simulink model "Interpretation_Unit"  (R2019a)
settings: Solver=ode2  StartTime=0.0  StopTime=inf  FixedStep=0.002  RelTol=1e-3  EnableMultiTasking=on
libraries: simulink x10, quarc_library x4
settings Model: Creator=User  LastModifiedBy=mbohra
settings SolverCC: PositivePriorityOrder=on
settings DataIOCC: ReturnWorkspaceOutputs=off
settings DebuggingCC: PregeneratedLibrarySubsystemCodeDiagnostic=none  ArithmeticOperatorsInVariantConditions=warning
settings SFSimCC: SimUseLocalCustomCode=off
settings RTWCC: SystemTargetFile=quarc_linux_nvidia.tlc  TemplateMakefile=quarc_linux_nvidia_tmf  Description=QUARC Linux Nvidia Target  RTWUseLocalCustomCode=off
settings STFCustomTargetCC: TargetLibSuffix=.a  TargetPreCompLibLocation=C:\PROGRA~3\QUARC\lib\2019a\LINUX_~1\release  TargetLangStandard=C99 (ISO)  ConcurrentExecutionCompliant=on  SystemTargetFile=quarc_linux_nvidia.tlc
settings GRTTargetCC: TargetLibSuffix=.a  TargetPreCompLibLocation=C:\PROGRA~3\QUARC\lib\2019a\LINUX_~1\release  ParMdlRefBuildCompliant=off  CompOptLevelCompliant=off  CombineOutputUpdateFcns=off  MatFileLogging=off  CPPClassGenCompliant=off  GRTInterface=on  UseToolchainInfoCompliant=off  ExtMode=on  ExtModeMexFile=quarc_comm  ExtModeMexArgs='-w -d /tmp -uri %u'

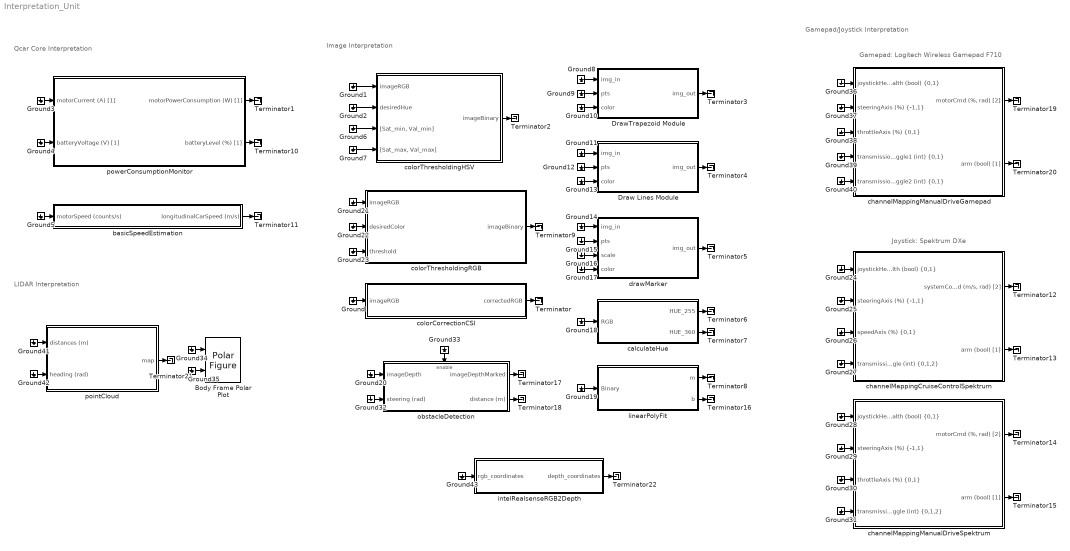
== system Interpretation_Unit ==
  note: LIDAR Interpretation
  note: Gamepad/Joystick Interpretation
  note: Image Interpretation
  note: Qcar Core Interpretation
  note: Gamepad: Logitech Wireless Gamepad F710
  note: Joystick: Spektrum DXe
  Body Frame Polar Plot : quarc_library/Sinks/Figures/Polar Figure  figure_mode=Use figure window  figure_tag=figure1  axes_tag=axes1  plot_mode=Frame-based  minimum_rho=0  maximum_rho=1  minimum_theta=0  maximum_theta=360  zero_location=right  direction=counterclockwise  buffer_size=1000  update_rate=1  sample_time=-1  initial_position="-1919             41           1920          990.4"  initial_visibility=off  line1_style=None  line1_width=0.5  line1_color=[0 0.4470 0.7410]  marker1=Circle (o)  marker1_size=1  marker1_edge_color=[0 0.447059 0.741176]  marker1_face_color=[0 0.447059 0.741176]  line2_style=Solid line (-)  line2_width=0.5  line2_color=[0.85098 0.32549 0.0980392]  marker2=None  marker2_size=6  marker2_edge_color=[0.85098 0.32549 0.0980392]  marker2_face_color=[0.85098 0.32549 0.0980392]  line3_style=Solid line (-)  line3_width=0.5  line3_color=[0.929412 0.694118 0.12549]  marker3=None  marker3_size=6  marker3_edge_color=[0.929412 0.694118 0.12549]  marker3_face_color=[0.929412 0.694118 0.12549]  line4_style=Solid line (-)  line4_width=0.5  line4_color=[0.494118 0.184314 0.556863]  marker4=None  marker4_size=6  marker4_edge_color=[0.494118 0.184314 0.556863]  marker4_face_color=[0.494118 0.184314 0.556863]  line5_style=Solid line (-)  line5_width=0.5  line5_color=[0.466667 0.67451 0.188235]  marker5=None  marker5_size=6  marker5_edge_color=[0.466667 0.67451 0.188235]  marker5_face_color=[0.466667 0.67451 0.188235]
      settings: SourceProductName=QUARC Targets
  Draw Lines Module : MATLAB Function  TreatAsAtomicUnit=on
  DrawTrapezoid Module : MATLAB Function  TreatAsAtomicUnit=on
  Ground{,1..43} (44 alike) : Ground
  Terminator{,1..22} (23 alike) : Terminator
  basicSpeedEstimation : Subsystem
  calculateHue : MATLAB Function  TreatAsAtomicUnit=on
  channelMappingCruiseControlSpektrum : Subsystem
  channelMappingManualDriveGamepad : Subsystem
  channelMappingManualDriveSpektrum : Subsystem
  colorCorrectionCSI : Subsystem
  colorThresholdingHSV : Subsystem
  colorThresholdingRGB : Subsystem
  drawMarker : MATLAB Function  TreatAsAtomicUnit=on
  intelRealsenseRGB2Depth : MATLAB Function  TreatAsAtomicUnit=on
  linearPolyFit : MATLAB Function  TreatAsAtomicUnit=on
  obstacleDetection : Subsystem
  pointCloud : Subsystem
  powerConsumptionMonitor : Subsystem
  wires:
  Ground23/1 -> colorThresholdingRGB/3("threshold ")
  basicSpeedEstimation/1(longitudinalCarSpeed (m/s)) -> Terminator11/1
  Ground18/1 -> calculateHue/1(RGB)
  calculateHue/1(HUE_255) -> Terminator6/1
  Ground22/1 -> colorThresholdingRGB/2(desiredColor)
  Ground5/1 -> basicSpeedEstimation/1(motorSpeed (counts/s))
  Ground1/1 -> colorThresholdingHSV/1(imageRGB)
  Ground8/1 -> DrawTrapezoid Module/1(img_in)
  Ground3/1 -> powerConsumptionMonitor/1(motorCurrent (A) [1])
  Ground14/1 -> drawMarker/1(img_in)
  Ground11/1 -> Draw Lines Module/1(img_in)
  Ground13/1 -> Draw Lines Module/3(color)
  powerConsumptionMonitor/2(batteryLevel (%) [1]) -> Terminator10/1
  colorThresholdingHSV/1(imageBinary) -> Terminator2/1
  powerConsumptionMonitor/1(motorPowerConsumption (W) [1]) -> Terminator1/1
  Ground16/1 -> drawMarker/3(scale)
  Ground7/1 -> colorThresholdingHSV/4("[Sat_max, Val_max]")
  Ground9/1 -> DrawTrapezoid Module/2(pts)
  Ground2/1 -> colorThresholdingHSV/2(desiredHue)
  Ground10/1 -> DrawTrapezoid Module/3(color)
  Ground15/1 -> drawMarker/2(pts)
  Ground12/1 -> Draw Lines Module/2(pts)
  Ground4/1 -> powerConsumptionMonitor/2(batteryVoltage (V) [1])
  Draw Lines Module/1(img_out) -> Terminator4/1
  colorThresholdingRGB/1(imageBinary) -> Terminator9/1
  Ground21/1 -> colorThresholdingRGB/1(imageRGB)
  DrawTrapezoid Module/1(img_out) -> Terminator3/1
  drawMarker/1(img_out) -> Terminator5/1
  colorCorrectionCSI/1(correctedRGB) -> Terminator/1
  Ground6/1 -> colorThresholdingHSV/3("[Sat_min, Val_min]")
  Ground17/1 -> drawMarker/4(color)
  calculateHue/2(HUE_360) -> Terminator7/1
  Ground/1 -> colorCorrectionCSI/1(imageRGB)
  channelMappingManualDriveSpektrum/2(arm (bool) [1]) -> Terminator15/1
  Ground25/1 -> channelMappingCruiseControlSpektrum/2("steeringAxis (%) {-1,1}")
  channelMappingCruiseControlSpektrum/2(arm (bool) [1]) -> Terminator13/1
  Ground29/1 -> channelMappingManualDriveSpektrum/2("steeringAxis (%) {-1,1}")
  channelMappingManualDriveSpektrum/1("motorCmd (%, rad) [2]") -> Terminator14/1
  Ground27/1 -> channelMappingCruiseControlSpektrum/4("transmissionToggle (int) {0,1,2}")
  Ground30/1 -> channelMappingManualDriveSpektrum/3("throttleAxis (%) {0,1}")
  Ground26/1 -> channelMappingCruiseControlSpektrum/3("speedAxis (%) {0,1}")
  Ground28/1 -> channelMappingManualDriveSpektrum/1("joystickHealth (bool) {0,1}")
  channelMappingCruiseControlSpektrum/1("systemCommand (m/s, rad) [2]") -> Terminator12/1
  Ground31/1 -> channelMappingManualDriveSpektrum/4("transmissionToggle (int) {0,1,2}")
  Ground24/1 -> channelMappingCruiseControlSpektrum/1("joystickHealth (bool) {0,1}")
  Ground34/1 -> Body Frame Polar Plot/1
  Ground35/1 -> Body Frame Polar Plot/2
  Ground36/1 -> channelMappingManualDriveGamepad/1("joystickHealth (bool) {0,1}")
  Ground37/1 -> channelMappingManualDriveGamepad/2("steeringAxis (%) {-1,1}")
  Ground38/1 -> channelMappingManualDriveGamepad/3("throttleAxis (%) {0,1}")
  Ground39/1 -> channelMappingManualDriveGamepad/4("transmissionToggle1 (int) {0,1}")
  Ground40/1 -> channelMappingManualDriveGamepad/5("transmissionToggle2 (int) {0,1}")
  channelMappingManualDriveGamepad/1("motorCmd (%, rad) [2]") -> Terminator19/1
  channelMappingManualDriveGamepad/2(arm (bool) [1]) -> Terminator20/1
  Ground41/1 -> pointCloud/1(distances (m))
  Ground42/1 -> pointCloud/2(heading (rad))
  pointCloud/1(map) -> Terminator21/1
  Ground19/1 -> linearPolyFit/1(Binary)
  linearPolyFit/1(m) -> Terminator8/1
  linearPolyFit/2(b) -> Terminator16/1
  Ground20/1 -> obstacleDetection/1(imageDepth)
  Ground32/1 -> obstacleDetection/2(steering (rad))
  obstacleDetection/1(imageDepthMarked) -> Terminator17/1
  obstacleDetection/2(distance (m)) -> Terminator18/1
  Ground33/1 -> obstacleDetection/Enable
  Ground43/1 -> intelRealsenseRGB2Depth/1(rgb_coordinates)
  intelRealsenseRGB2Depth/1(depth_coordinates) -> Terminator22/1

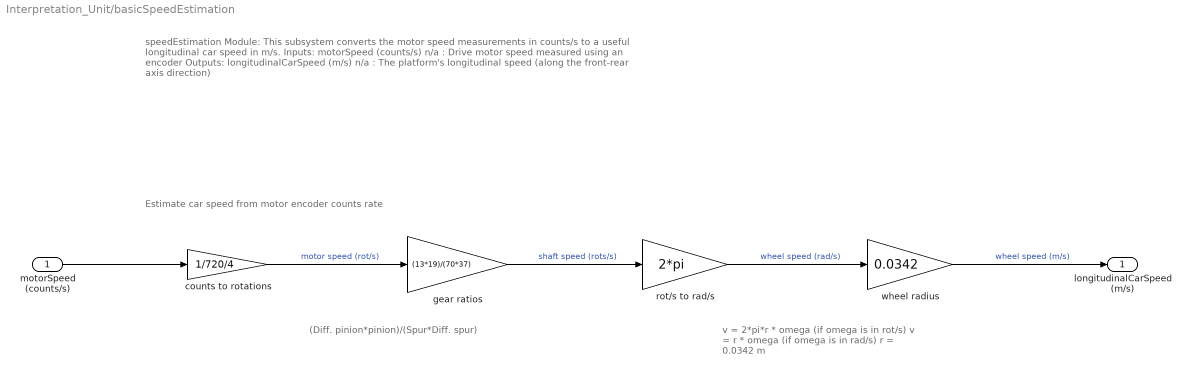
== system Interpretation_Unit/basicSpeedEstimation ==
  note: Estimate car speed from motor encoder counts rate
  note: v = 2*pi*r * omega (if omega is in rot/s)
      | v = r * omega (if omega is in rad/s)
      | r = 0.0342 m
  note: (Diff. pinion*pinion)/(Spur*Diff. spur)
  note: speedEstimation Module:
      |
      | This subsystem converts the motor speed measurements in counts/s to a useful longitudinal car speed in m/s.
      |
      | Inputs:
      | motorSpeed (counts/s) n/a : Drive motor speed measured using an encoder
      |
      | Outputs:
      | longitudinalCarSpeed (m/s) n/a : The platform's longitudinal speed (along the front-rear axis direction)
  motorSpeed (counts/s) : Inport
  counts to rotations : Gain  Gain=1/720/4
  gear ratios : Gain  Gain=(13*19)/(70*37)
  rot/s to rad/s : Gain  Gain=2*pi
  wheel radius : Gain  Gain=0.0342
  longitudinalCarSpeed (m/s) : Outport
  wires:
  motorSpeed (counts/s)/1 -> counts to rotations/1
  rot/s to rad/s/1 -> wheel radius/1  "wheel speed (rad/s)"
  counts to rotations/1 -> gear ratios/1  "motor speed (rot/s)"
  wheel radius/1 -> longitudinalCarSpeed (m/s)/1  "wheel speed (m/s)"
  gear ratios/1 -> rot/s to rad/s/1  "shaft speed (rots/s)"

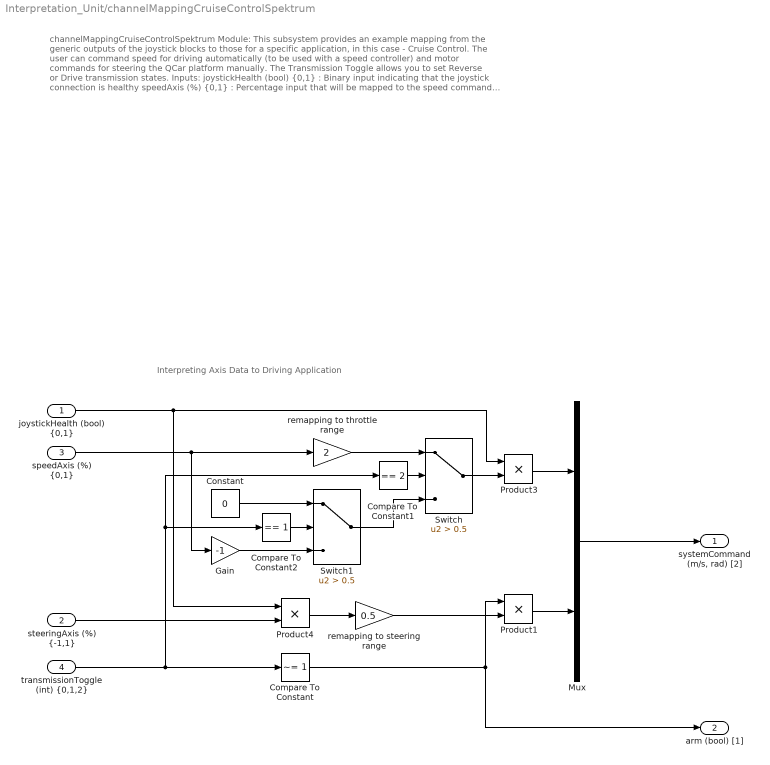
== system Interpretation_Unit/channelMappingCruiseControlSpektrum ==
  note: Interpreting Axis Data to Driving Application
  note: channelMappingCruiseControlSpektrum Module:
      |
      | This subsystem provides an example mapping from the generic outputs of the joystick blocks to those for a specific application, in this case - Cruise Control. The user can command speed for driving automatically (to be used with a speed controller) and motor commands for steering the QCar platform manually. The Transmission Toggle allows you to set Reverse or Drive transmission states.
      |
      | Inputs:
      | joystickHealth (bool) {0,1} : Binary input indicating that the joystick connection is healthy
      | speedAxis (%) {0,1} : Percentage input that will be mapped to the speed command
      | steeringAxis (%) {-1,1} : Signed percentage input that will be mapped to steering
      | transmissionToggle (int) {0,1,2} : 3-state input that will decide the Reverse/Park/Drive states
      |
      | Outputs:
      | systemCommand (m/s, rad) n/a : Vector output for the speed command (m/s) as well as steering command (in rad)
      | arm (bool) {0,1} : Binary output indicating status (armed or disarmed)
      |
      | Usage:
      | 1. When the Transmission Toggle input
      | a. reads 0 or 2, the Arm output will be high (1), which is the Armed state.
      | b. reads 1, the Arm output will be low (0), which is the Disarmed state.
      | 2. In addition, the Transmission Toggle input
      | a. reading 0 is the Reverse state, and the Speed Command will range from 0 m/s to -1 m/s, spinning the wheels backwards.
      | b. reading 1 is the Park state, and the Speed Command will be zero.
      | c. reading 2 is the Drive state, and the Speed Command will range from 0 m/s to 2 m/s, spinning the wheels forwards.
  "joystickHealth (bool) {0,1}" : Inport
  "steeringAxis (%) {-1,1}" : Inport  Port=2
  "speedAxis (%) {0,1}" : Inport  Port=3
  "transmissionToggle (int) {0,1,2}" : Inport  Port=4
  " remapping to steering range " : Gain  Gain=0.5
  Compare To Constant : simulink/Logic and Bit Operations/Compare To Constant  relop=~=  const=1  OutDataTypeStr=boolean
  Compare To Constant1 : simulink/Logic and Bit Operations/Compare To Constant  relop===  const=2  OutDataTypeStr=boolean
  Compare To Constant2 : simulink/Logic and Bit Operations/Compare To Constant  relop===  const=1  OutDataTypeStr=boolean
  Constant : Constant  Value=0
  Gain : Gain  Gain=-1
  Mux : Mux  Inputs=2
  Product1 : Product
  Product3 : Product
  Product4 : Product
  Switch : Switch  Criteria=u2 > Threshold  Threshold=0.5
  Switch1 : Switch  Criteria=u2 > Threshold  Threshold=0.5
  remapping to throttle range : Gain  Gain=2
  "systemCommand (m/s, rad) [2]" : Outport
  arm (bool) [1] : Outport  Port=2
  wires:
  Switch1/1 -> Switch/3
  Gain/1 -> Switch1/3
  Compare To Constant/1 -> arm (bool) [1]/1, Product1/1
  Compare To Constant2/1 -> Switch1/2
  Constant/1 -> Switch1/1
  "joystickHealth (bool) {0,1}"/1 -> Product3/1, Product4/1
  Compare To Constant1/1 -> Switch/2
  Product4/1 -> " remapping to steering range "/1
  remapping to throttle range/1 -> Switch/1
  "transmissionToggle (int) {0,1,2}"/1 -> Compare To Constant2/1, Compare To Constant1/1, Compare To Constant/1
  Product3/1 -> Mux/1
  "speedAxis (%) {0,1}"/1 -> Gain/1, remapping to throttle range/1
  " remapping to steering range "/1 -> Product1/2
  "steeringAxis (%) {-1,1}"/1 -> Product4/2
  Product1/1 -> Mux/2
  Mux/1 -> "systemCommand (m/s, rad) [2]"/1
  Switch/1 -> Product3/2

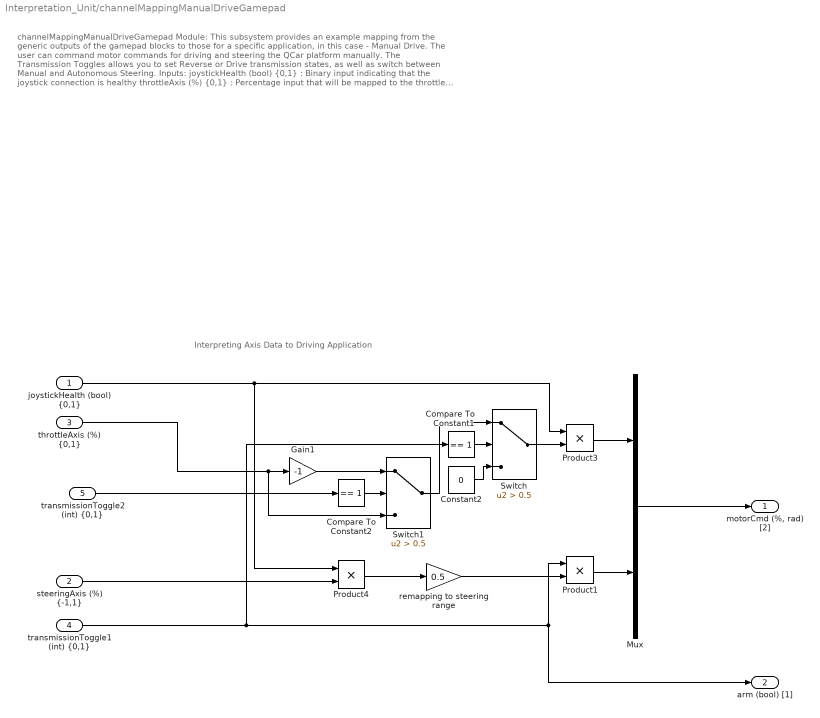
== system Interpretation_Unit/channelMappingManualDriveGamepad ==
  note: Interpreting Axis Data to Driving Application
  note: channelMappingManualDriveGamepad Module:
      |
      | This subsystem provides an example mapping from the generic outputs of the gamepad blocks to those for a specific application, in this case - Manual Drive. The user can command motor commands for driving and steering the QCar platform manually. The Transmission Toggles allows you to set Reverse or Drive transmission states, as well as switch between Manual and Autonomous Steering.
      |
      | Inputs:
      | joystickHealth (bool) {0,1} : Binary input indicating that the joystick connection is healthy
      | throttleAxis (%) {0,1} : Percentage input that will be mapped to the throttle command
      | steeringAxis (%) {-1,1} : Signed percentage input that will be mapped to steering
      | transmissionToggle1 (int) {0,1} : 2-state input that will decide the Park/Engage State
      | transmissionToggle2 (int) {0, 1} : 2-state input that will decide the Reverse/Drive State
      |
      | Outputs:
      | motorCmd (%, rad) n/a : Vector output for the motor drive command (percentage throttle) as well as steering command (in rad)
      | arm (bool) {0,1} : Binary output indicating status (armed or disarmed)
      |
      | Usage:
      | 1. When the Transmission Toggle 1 input
      | a. reads 1, the Arm output will be high (1), which is the Armed state.
      | b. reads 0, the Arm output will be low (0), which is the Disarmed state.
      | 2. In addition, the Transmission Toggle 2 input
      | a. reading 0 is the Drive state, and the Motor Cmd for the throttle will range from 0 to 100%, spinning the wheels forwards.
      | b. reading 1 is the Reverse state, and the Motor Cmd for the throttle will range from 0 to -100%, spinning the wheels backwards.
  "joystickHealth (bool) {0,1}" : Inport
  "steeringAxis (%) {-1,1}" : Inport  Port=2
  "throttleAxis (%) {0,1}" : Inport  Port=3
  "transmissionToggle1 (int) {0,1}" : Inport  Port=4
  "transmissionToggle2 (int) {0,1}" : Inport  Port=5
  " remapping to steering range " : Gain  Gain=0.5
  Compare To Constant1 : simulink/Logic and Bit Operations/Compare To Constant  relop===  const=1  OutDataTypeStr=boolean
  Compare To Constant2 : simulink/Logic and Bit Operations/Compare To Constant  relop===  const=1  OutDataTypeStr=boolean
  Constant2 : Constant  Value=0
  Gain1 : Gain  Gain=-1
  Mux : Mux  Inputs=2
  Product1 : Product
  Product3 : Product
  Product4 : Product
  Switch : Switch  Criteria=u2 > Threshold  Threshold=0.5
  Switch1 : Switch  Criteria=u2 > Threshold  Threshold=0.5
  "motorCmd (%, rad) [2]" : Outport
  arm (bool) [1] : Outport  Port=2
  wires:
  Gain1/1 -> Switch1/1
  "transmissionToggle2 (int) {0,1}"/1 -> Compare To Constant2/1
  Constant2/1 -> Switch/3
  Switch1/1 -> Switch/1
  Compare To Constant2/1 -> Switch1/2
  Mux/1 -> "motorCmd (%, rad) [2]"/1
  "throttleAxis (%) {0,1}"/1 -> Gain1/1, Switch1/3
  Product4/1 -> " remapping to steering range "/1
  " remapping to steering range "/1 -> Product1/2
  Product3/1 -> Mux/1
  "transmissionToggle1 (int) {0,1}"/1 -> arm (bool) [1]/1, Product1/1, Compare To Constant1/1
  "joystickHealth (bool) {0,1}"/1 -> Product3/1, Product4/1
  "steeringAxis (%) {-1,1}"/1 -> Product4/2
  Compare To Constant1/1 -> Switch/2
  Product1/1 -> Mux/2
  Switch/1 -> Product3/2

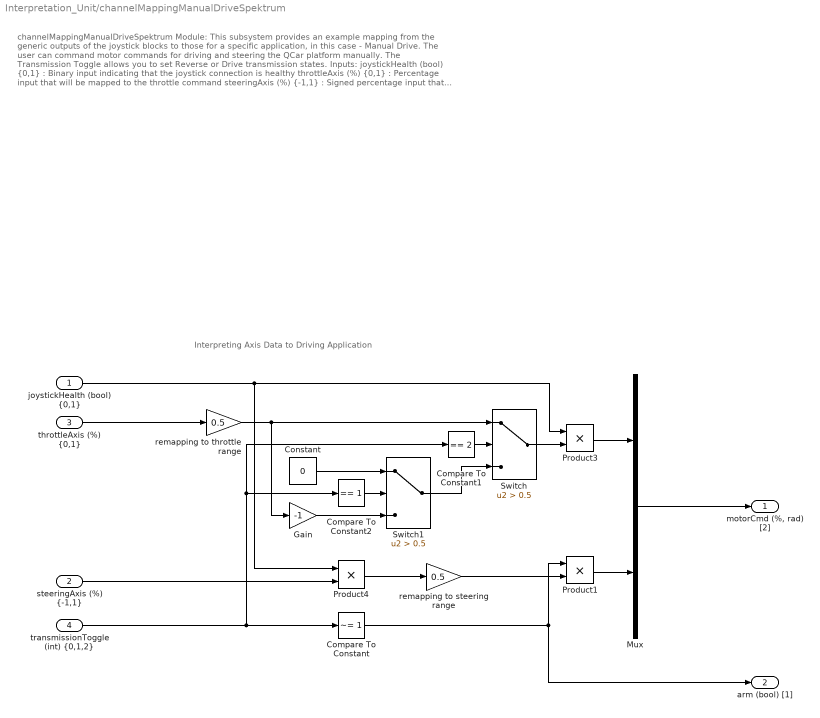
== system Interpretation_Unit/channelMappingManualDriveSpektrum ==
  note: Interpreting Axis Data to Driving Application
  note: channelMappingManualDriveSpektrum Module:
      |
      | This subsystem provides an example mapping from the generic outputs of the joystick blocks to those for a specific application, in this case - Manual Drive. The user can command motor commands for driving and steering the QCar platform manually. The Transmission Toggle allows you to set Reverse or Drive transmission states.
      |
      | Inputs:
      | joystickHealth (bool) {0,1} : Binary input indicating that the joystick connection is healthy
      | throttleAxis (%) {0,1} : Percentage input that will be mapped to the throttle command
      | steeringAxis (%) {-1,1} : Signed percentage input that will be mapped to steering
      | transmissionToggle (int) {0,1,2} : 3-state input that will decide the Reverse/Park/Drive states
      |
      | Outputs:
      | motorCmd (%, rad) n/a : Vector output for the motor drive command (percentage throttle) as well as steering command (in rad)
      | arm (bool) {0,1} : Binary output indicating status (armed or disarmed)
      |
      | Usage:
      | 1. When the Transmission Toggle input
      | a. reads 0 or 2, the Arm output will be high (1), which is the Armed state.
      | b. reads 1, the Arm output will be low (0), which is the Disarmed state.
      | 2. In addition, the Transmission Toggle input
      | a. reading 0 is the Reverse state, and the Motor Cmd for the throttle will range from 0 to -50%, spinning the wheels backwards.
      | b. reading 1 is the Park state, and the Motor Cmd for the throttle will be zero.
      | c. reading 2 is the Drive state, and the Motor Cmd for the throttle will range from 0 to 50%, spinning the wheels forwards.
  "joystickHealth (bool) {0,1}" : Inport
  "steeringAxis (%) {-1,1}" : Inport  Port=2
  "throttleAxis (%) {0,1}" : Inport  Port=3
  "transmissionToggle (int) {0,1,2}" : Inport  Port=4
  " remapping to steering range " : Gain  Gain=0.5
  " remapping to throttle range" : Gain  Gain=0.5
  Compare To Constant : simulink/Logic and Bit Operations/Compare To Constant  relop=~=  const=1  OutDataTypeStr=boolean
  Compare To Constant1 : simulink/Logic and Bit Operations/Compare To Constant  relop===  const=2  OutDataTypeStr=boolean
  Compare To Constant2 : simulink/Logic and Bit Operations/Compare To Constant  relop===  const=1  OutDataTypeStr=boolean
  Constant : Constant  Value=0
  Gain : Gain  Gain=-1
  Mux : Mux  Inputs=2
  Product1 : Product
  Product3 : Product
  Product4 : Product
  Switch : Switch  Criteria=u2 > Threshold  Threshold=0.5
  Switch1 : Switch  Criteria=u2 > Threshold  Threshold=0.5
  "motorCmd (%, rad) [2]" : Outport
  arm (bool) [1] : Outport  Port=2
  wires:
  " remapping to throttle range"/1 -> Switch/1, Gain/1
  Constant/1 -> Switch1/1
  Compare To Constant2/1 -> Switch1/2
  Mux/1 -> "motorCmd (%, rad) [2]"/1
  Gain/1 -> Switch1/3
  Product4/1 -> " remapping to steering range "/1
  " remapping to steering range "/1 -> Product1/2
  Product3/1 -> Mux/1
  Compare To Constant/1 -> arm (bool) [1]/1, Product1/1
  "throttleAxis (%) {0,1}"/1 -> " remapping to throttle range"/1
  Switch1/1 -> Switch/3
  "joystickHealth (bool) {0,1}"/1 -> Product3/1, Product4/1
  "steeringAxis (%) {-1,1}"/1 -> Product4/2
  Compare To Constant1/1 -> Switch/2
  "transmissionToggle (int) {0,1,2}"/1 -> Compare To Constant2/1, Compare To Constant1/1, Compare To Constant/1
  Product1/1 -> Mux/2
  Switch/1 -> Product3/2

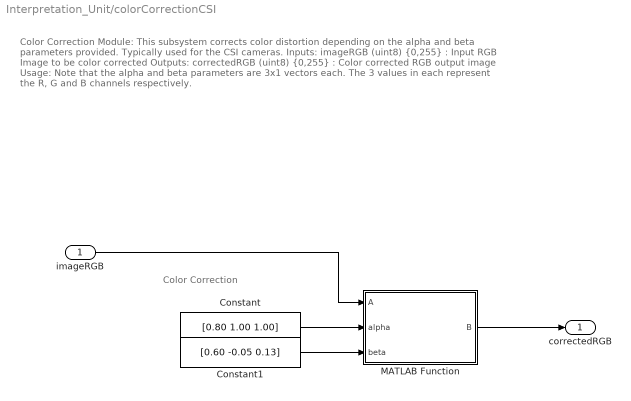
== system Interpretation_Unit/colorCorrectionCSI ==
  note: Color Correction
  note: Color Correction Module:
      |
      | This subsystem corrects color distortion depending on the alpha and beta parameters provided. Typically used for the CSI cameras.
      |
      | Inputs:
      | imageRGB (uint8) {0,255} : Input RGB Image to be color corrected
      |
      | Outputs:
      | correctedRGB (uint8) {0,255} : Color corrected RGB output image
      |
      | Usage:
      | Note that the alpha and beta parameters are 3x1 vectors each. The 3 values in each represent the R, G and B channels respectively.
  imageRGB : Inport
  Constant : Constant  Value=[0.80 1.00 1.00]
  Constant1 : Constant  Value=[0.60 -0.05 0.13]
  MATLAB Function : MATLAB Function  TreatAsAtomicUnit=on
  correctedRGB : Outport
  wires:
  Constant1/1 -> MATLAB Function/3(beta)
  MATLAB Function/1(B) -> correctedRGB/1
  imageRGB/1 -> MATLAB Function/1(A)
  Constant/1 -> MATLAB Function/2(alpha)

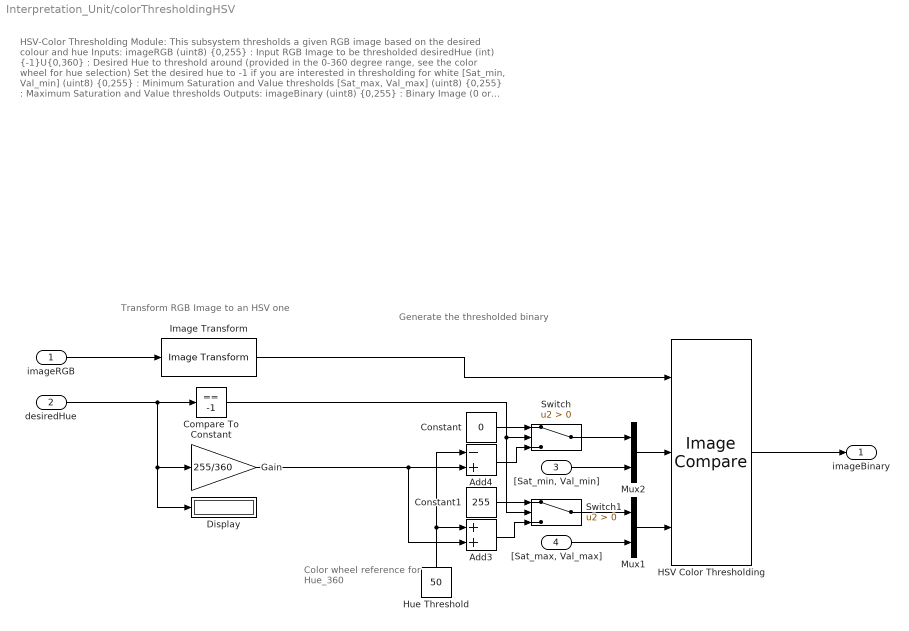
== system Interpretation_Unit/colorThresholdingHSV ==
  note: Generate the thresholded binary
  note: Transform RGB Image to an HSV one
  note: Color wheel
      | reference
      | for Hue_360
  note: HSV-Color Thresholding Module:
      |
      | This subsystem thresholds a given RGB image based on the desired colour and hue
      |
      | Inputs:
      | imageRGB (uint8) {0,255} : Input RGB Image to be thresholded
      | desiredHue (int) {-1}U{0,360} : Desired Hue to threshold around (provided in the 0-360 degree range, see the color wheel for hue selection)
      | Set the desired hue to -1 if you are interested in thresholding for white
      | [Sat_min, Val_min] (uint8) {0,255} : Minimum Saturation and Value thresholds
      | [Sat_max, Val_max] (uint8) {0,255} : Maximum Saturation and Value thresholds
      |
      | Outputs:
      | imageBinary (uint8) {0,255} : Binary Image (0 or 255 and no other value) representing the thresholding output
      |
      | Usage:
      | This module can be used when you are interested in thresholding for a certain hue regardless of the luminance. Compared to RGB thresholding which does not work well when the lighting conditions vary, HSV thresholding will correctly threshold for a hue (color) and allow you to specify a broad range of illuminance via the saturation and value thresholds. To broaden the range of hues accepted in the thresholding block, increase the Hue Threshold parameter.
  imageRGB : Inport
  desiredHue : Inport  Port=2
  "[Sat_min, Val_min]" : Inport  Port=3
  "[Sat_max, Val_max]" : Inport  Port=4
  Add3 : Sum
  Add4 : Sum  Inputs=-+
  Compare To Constant : simulink/Logic and Bit Operations/Compare To Constant  relop===  const=-1  OutDataTypeStr=boolean
  Constant : Constant  Value=0
  Constant1 : Constant  Value=255
  Display : Display
  Gain : Gain  Gain=255/360
  HSV Color Thresholding : quarc_library/Image Processing/Generic/Image Compare  output_type=Combined (one HxW output)  source=External input ports  r_comparison=min <= pixel and pixel <= max with wrapping  r_minimum=30  r_maximum=70  g_comparison=min <= pixel and pixel <= max  g_minimum=60  g_maximum=100  b_comparison=min <= pixel and pixel <= max  b_minimum=40  b_maximum=80
      settings: SourceProductName=QUARC Targets
  Hue Threshold : Constant  Value=50
  Image Transform : quarc_library/Image Processing/Generic/Image Transform  algorithm=RGB to HSV  color_theme=KRYGCBMW  min_pixel=0  max_pixel=4000
      settings: AttributesFormatString=(%<algorithm>)  SourceProductName=QUARC Targets
  Mux1 : Mux  Inputs=2
  Mux2 : Mux  Inputs=2
  Switch : Switch  Criteria=u2 > Threshold
  Switch1 : Switch  Criteria=u2 > Threshold
  imageBinary : Outport
  wires:
  imageRGB/1 -> Image Transform/1
  Hue Threshold/1 -> Add3/1, Add4/1
  Image Transform/1 -> HSV Color Thresholding/1
  desiredHue/1 -> Compare To Constant/1, Display/1, Gain/1
  Gain/1 -> Add4/2, Add3/2
  Constant1/1 -> Switch1/1
  "[Sat_max, Val_max]"/1 -> Mux1/2
  Add3/1 -> Switch1/3
  Switch/1 -> Mux2/1
  Compare To Constant/1 -> Switch/2, Switch1/2
  Constant/1 -> Switch/1
  Switch1/1 -> Mux1/1
  Mux1/1 -> HSV Color Thresholding/3
  Add4/1 -> Switch/3
  "[Sat_min, Val_min]"/1 -> Mux2/2
  Mux2/1 -> HSV Color Thresholding/2
  HSV Color Thresholding/1 -> imageBinary/1

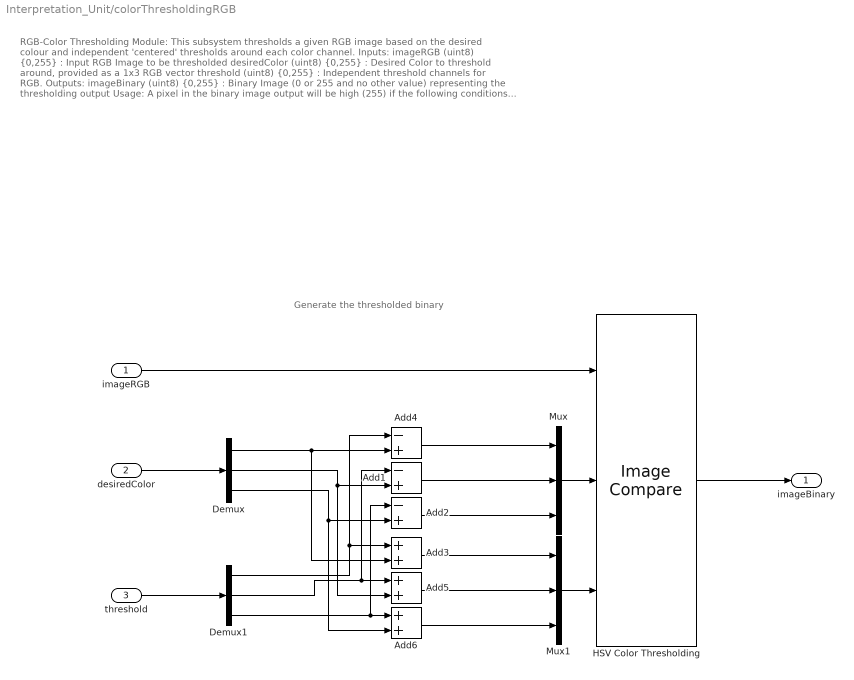
== system Interpretation_Unit/colorThresholdingRGB ==
  note: RGB-Color Thresholding Module:
      |
      | This subsystem thresholds a given RGB image based on the desired colour and independent 'centered' thresholds around each color channel.
      |
      | Inputs:
      | imageRGB (uint8) {0,255} : Input RGB Image to be thresholded
      | desiredColor (uint8) {0,255} : Desired Color to threshold around, provided as a 1x3 RGB vector
      | threshold (uint8) {0,255} : Independent threshold channels for RGB.
      |
      | Outputs:
      | imageBinary (uint8) {0,255} : Binary Image (0 or 255 and no other value) representing the thresholding output
      |
      | Usage:
      | A pixel in the binary image output will be high (255) if the following conditions are met for the same pixel in the red, blue and green planes of the input image
      | ( red_value >= desired_color_red - red_threshold AND red_value <= desired_color_red + red_threshold ), AND
      | ( green_value >= desired_color_green - green_threshold AND green_value <= desired_color_green + green_threshold ), AND
      | ( blue_value >= desired_color_blue - blue_threshold AND blue_value <= desired_color_blue + blue_threshold )
  note: Generate the thresholded binary
  imageRGB : Inport
  desiredColor : Inport  Port=2
  "threshold " : Inport  Port=3
  Add1 : Sum  Inputs=-+
  Add2 : Sum  Inputs=-+
  Add3 : Sum
  Add4 : Sum  Inputs=-+
  Add5 : Sum
  Add6 : Sum
  Demux : Demux  Outputs=3
  Demux1 : Demux  Outputs=3
  HSV Color Thresholding : quarc_library/Image Processing/Generic/Image Compare  output_type=Combined (one HxW output)  source=External input ports  r_comparison=min <= pixel and pixel <= max  r_minimum=30  r_maximum=70  g_comparison=min <= pixel and pixel <= max  g_minimum=60  g_maximum=100  b_comparison=min <= pixel and pixel <= max  b_minimum=40  b_maximum=80
      settings: SourceProductName=QUARC Targets
  Mux : Mux  Inputs=3
  Mux1 : Mux  Inputs=3
  imageBinary : Outport
  wires:
  Mux1/1 -> HSV Color Thresholding/3
  Demux/1 -> Add3/2, Add4/2
  imageRGB/1 -> HSV Color Thresholding/1
  Add5/1 -> Mux1/2
  Add6/1 -> Mux1/3
  desiredColor/1 -> Demux/1
  Demux1/3 -> Add2/1, Add6/1
  Demux1/1 -> Add4/1, Add3/1
  Add2/1 -> Mux/3
  Add3/1 -> Mux1/1
  HSV Color Thresholding/1 -> imageBinary/1
  Add1/1 -> Mux/2
  Mux/1 -> HSV Color Thresholding/2
  Demux1/2 -> Add1/1, Add5/1
  Add4/1 -> Mux/1
  "threshold "/1 -> Demux1/1
  Demux/3 -> Add2/2, Add6/2
  Demux/2 -> Add1/2, Add5/2

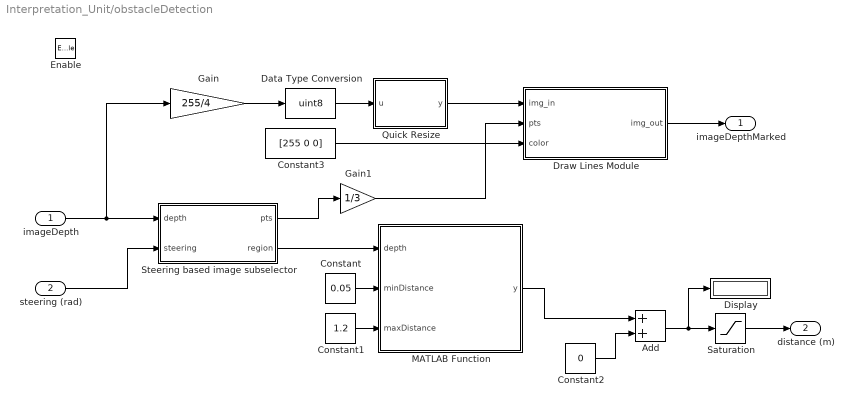
== system Interpretation_Unit/obstacleDetection ==
  imageDepth : Inport
  steering (rad) : Inport  Port=2
  Enable : EnablePort  PropagateVarSize=During execution
  Add : Sum
  Constant : Constant  Value=0.05
  Constant1 : Constant  Value=1.2
  Constant2 : Constant  Value=0
  Constant3 : Constant  Value=[255 0 0]
  Data Type Conversion : DataTypeConversion  OutDataTypeStr=uint8
  Display : Display
  Draw Lines Module : MATLAB Function  TreatAsAtomicUnit=on
  Gain : Gain  Gain=255/4
  Gain1 : Gain  Gain=1/3
  MATLAB Function : MATLAB Function  TreatAsAtomicUnit=on
  Quick Resize : MATLAB Function  TreatAsAtomicUnit=on
  Saturation : Saturate  UpperLimit=1.2  LowerLimit=0.2
  Steering based image subselector : MATLAB Function  TreatAsAtomicUnit=on
  imageDepthMarked : Outport
  distance (m) : Outport  Port=2
  wires:
  Draw Lines Module/1(img_out) -> imageDepthMarked/1
  Gain1/1 -> Draw Lines Module/2(pts)
  Data Type Conversion/1 -> Quick Resize/1(u)
  Quick Resize/1(y) -> Draw Lines Module/1(img_in)
  Gain/1 -> Data Type Conversion/1
  imageDepth/1 -> Gain/1, Steering based image subselector/1(depth)
  MATLAB Function/1(y) -> Add/1
  Constant/1 -> MATLAB Function/2(minDistance)
  Constant1/1 -> MATLAB Function/3(maxDistance)
  Constant2/1 -> Add/2
  Add/1 -> Saturation/1, Display/1
  Saturation/1 -> distance (m)/1
  steering (rad)/1 -> Steering based image subselector/2(steering)
  Steering based image subselector/2(region) -> MATLAB Function/1(depth)
  Steering based image subselector/1(pts) -> Gain1/1
  Constant3/1 -> Draw Lines Module/3(color)

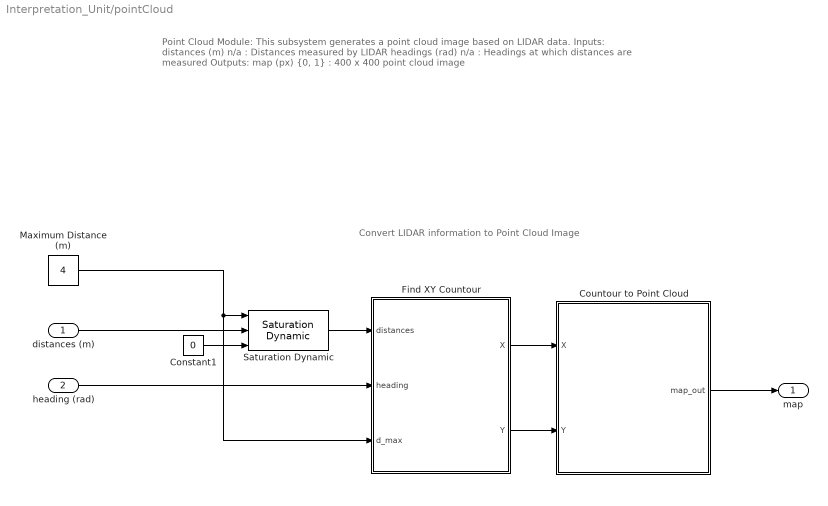
== system Interpretation_Unit/pointCloud ==
  note: Point Cloud Module:
      |
      | This subsystem generates a point cloud image based on LIDAR data.
      |
      | Inputs:
      | distances (m) n/a : Distances measured by LIDAR
      | headings (rad) n/a : Headings at which distances are measured
      |
      | Outputs:
      | map (px) {0, 1} : 400 x 400 point cloud image
  note: Convert LIDAR information to Point Cloud Image
  distances (m) : Inport
  heading (rad) : Inport  Port=2
  Constant1 : Constant  Value=0
  Countour to Point Cloud : MATLAB Function  TreatAsAtomicUnit=on
  Find XY Countour : MATLAB Function  TreatAsAtomicUnit=on
  Maximum Distance (m) : Constant  Value=4
  Saturation Dynamic : simulink/Discontinuities/Saturation Dynamic  OutMin=[]  OutMax=[]  OutDataTypeStr=Inherit: Same as second input  OutDataType=fixdt(1, 16)  OutScaling=2^-10  DoSatur=off
  map : Outport
  wires:
  Find XY Countour/2(Y) -> Countour to Point Cloud/2(Y)
  Find XY Countour/1(X) -> Countour to Point Cloud/1(X)
  Constant1/1 -> Saturation Dynamic/3
  Maximum Distance (m)/1 -> Saturation Dynamic/1, Find XY Countour/3(d_max)
  Saturation Dynamic/1 -> Find XY Countour/1(distances)
  Countour to Point Cloud/1(map_out) -> map/1
  distances (m)/1 -> Saturation Dynamic/2
  heading (rad)/1 -> Find XY Countour/2(heading)

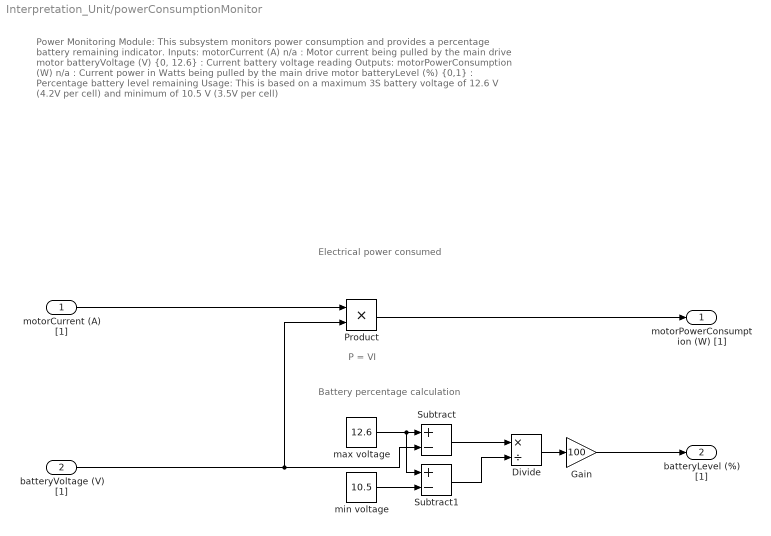
== system Interpretation_Unit/powerConsumptionMonitor ==
  note: Power Monitoring Module:
      |
      | This subsystem monitors power consumption and provides a percentage battery remaining indicator.
      |
      | Inputs:
      | motorCurrent (A) n/a : Motor current being pulled by the main drive motor
      | batteryVoltage (V) {0, 12.6} : Current battery voltage reading
      |
      | Outputs:
      | motorPowerConsumption (W) n/a : Current power in Watts being pulled by the main drive motor
      | batteryLevel (%) {0,1} : Percentage battery level remaining
      |
      | Usage:
      | This is based on a maximum 3S battery voltage of 12.6 V (4.2V per cell) and minimum of 10.5 V (3.5V per cell)
  note: Electrical
      | power
      | consumed
  note: P = VI
  note: Battery percentage calculation
  motorCurrent (A) [1] : Inport
  batteryVoltage (V) [1] : Inport  Port=2
  Divide : Product  Inputs=*/
  Gain : Gain  Gain=100
  Product : Product
  Subtract : Sum  Inputs=+-
  Subtract1 : Sum  Inputs=+-
  max voltage : Constant  Value=12.6
  min voltage : Constant  Value=10.5
  motorPowerConsumption (W) [1] : Outport
  batteryLevel (%) [1] : Outport  Port=2
  wires:
  batteryVoltage (V) [1]/1 -> Product/2, Subtract/2
  Subtract/1 -> Divide/1
  max voltage/1 -> Subtract1/1, Subtract/1
  motorCurrent (A) [1]/1 -> Product/1
  min voltage/1 -> Subtract1/2
  Product/1 -> motorPowerConsumption (W) [1]/1
  Gain/1 -> batteryLevel (%) [1]/1
  Subtract1/1 -> Divide/2
  Divide/1 -> Gain/1

== matlab function Interpretation_Unit/Draw Lines Module ==
  data: img_in input; img_out output; pts input; color input
function img_out = drawLines(img_in, pts, color)

% Draw lines connecting the points using the provided color

% Inputs:
% u         : Input RGB Image (size = m by n)
% pts       : p x-y pairs of points (px) where markers are to be drawn
% color     : 1x3 matrix of RGB color values for each marker

% Outputs:
% y         : Output RGB Image with the markers drawn in (size = m by n)

%% Initialization
img_out = img_in;
[p, ~] = size(pts); % determine the number of points

%% Draw the lines
    for i = 1:p-1
        % determine the max(rows_difference, col_difference) between two
        % points
        itr = max(abs(pts(i,1) - pts(i+1,1)), abs(pts(i,2) - pts(i+1,2)));
        
        % generate linear spaces of row and col values between the pts
        row_vec = round(linspace(pts(i,1), pts(i+1,1), itr));
        col_vec = round(linspace(pts(i,2), pts(i+1,2), itr));
        
        % iterate through the values and shade them right
        for j = 1:itr
            img_out(row_vec(j), col_vec(j),1) = color(1);
            img_out(row_vec(j), col_vec(j),2) = color(2);
            img_out(row_vec(j), col_vec(j),3) = color(3);
        end
    end
end

== matlab function Interpretation_Unit/DrawTrapezoid Module ==
  data: img_in input; img_out output; pts input; color input
function img_out  = drawTrapezoid(img_in, pts, color)

% Shade a trapezoid in the input image between the boundary points in the
% given color

% Inputs:
% u         : Input RGB Image (size = m by n)
% pts       : 4 x-y pairs of points (px) representing the vertices
%             Format: TL, TR, BL, BR 
% color     : 1x3 matrix of RGB color values for each marker

% Outputs:
% y         : Output RGB Image with the markers drawn in (size = m by n)

%% Initialization
img_out = img_in; % Initializes the output image to be modified
left_vertical = 0; % Assume the left line isn't vertical
right_vertical = 0; % Assume the right line isn't vertical

%% Left and Right lines
% Given: row_px = slope * col_px + intercept 
% determine slope of left edge line of trapezoid based on the first and third points
if (pts(1,2)== pts(3,2))
    left_vertical = 1;
    m_left = 1; % default value for a slope, becuase in this case, slope won't be used
else
    m_left = (pts(1,1)-pts(3,1))/(pts(1,2)-pts(3,2));
end

% determine the intercept of the left edge line of trapezoid from the first and third points
b_left = pts(1,1) - (m_left*pts(1,2));

% determine slope of the right edge line of trapezoid based on second and fourth points
if (pts(2,2)== pts(4,2))
    right_vertical = 1;
    m_right = 1; % default value for a slope, becuase in this case, slope won't be used
else
    m_right = (pts(2,1)-pts(4,1))/(pts(2,2)-pts(4,2));
end

% determine the intercept of the right edge line of trapezoid from the second and fourth points
b_right = pts(2,1) - (m_right*pts(2,2));

%% Shade the Trapezoid
    for i = pts(1,1):1:pts(3,1) 
    % iterate through the rows starting from the top row to the bottom one.
    % In each row, iterate through the cols from s (start) to
    % f (finish).  
        if left_vertical
            s = pts(1,2);
        else
            s = round((i-b_left)/m_left);   % function of m_left, b_left and i
        end
        
        if right_vertical
            f = pts(2,2);
        else
            f = round((i-b_right)/m_right); % function of m_right, b_right and i
        end
    
        img_out( i, s:f, 1) = color(1); % first color
        img_out( i, s:f, 2) = color(2); % second color
        img_out( i, s:f, 3) = color(3); % third color      
        
    end
    
end

== matlab function Interpretation_Unit/drawMarker ==
  data: img_in input; img_out output; pts input; scale input; color input
function img_out = drawMarker(img_in, pts, scale, color)

% Draw square markers at user defined locations

% Inputs:
% u         : Input RGB Image (size = m by n)
% pts       : qx2 x-y pairs of points (px) where markers are to be drawn
% scale     : qx1 vector (%) representing size of each marker w.r.t m
% color     : qx3 matrix of RGB color values for each marker

% Outputs:
% y         : Output RGB Image with the markers drawn in (size = m by n)

%% Initialization

img_out = img_in;

[m, ~] = size(img_in); % image size (m - rows, n - cols)
q = length(scale); % determine the number of points

%% Draw Markers
    for i = 1:q
        % determine the actual size of marker in pixels (side length / 2)
        p = round(scale(i)*m/2); 
        
        % draw the markers
        img_out( pts(i,1) - p : pts(i,1) + p,   pts(i,2) - p : pts(i,2) + p,   1 ) = color(i,1);
        img_out( pts(i,1) - p : pts(i,1) + p,   pts(i,2) - p : pts(i,2) + p,   2 ) = color(i,2);
        img_out( pts(i,1) - p : pts(i,1) + p,   pts(i,2) - p : pts(i,2) + p,   3 ) = color(i,3);
    end
end

== matlab function Interpretation_Unit/calculateHue ==
  data: RGB input; HUE_255 output; HUE_360 output
function [HUE_255, HUE_360]  = calculateHue(RGB)

% Calculates the HUE value corresponding to a desired RGB value
% Note that RGB specifies not only the color channels, but also a combined
% luminance or brightness. Thus, multiple RGB value pairs may result in the
% same hue, and this does not paint a complete picture. One must also
% consider the saturation and value parameters to uniquely relate RGB and
% HSV triplet pairs. 

% Inputs:
% RGB     :     R G and B values as desired
 
% Outputs:
% HUE_255 :     255 scale hue
% HUE_360 :     360 degree hue

%% Initialization
HUE = 0;

rgb = RGB./255;
[val_max, index_max] = max(rgb);
[val_min, ~] = min(rgb);
delta = val_max - val_min;

%% HUE
    if delta == 0 % delta being zero relates to the fact that the R, G and B
                  % values are equal. This will lead to a 0/0 case in the
                  % else case below.
        HUE = 0;
    else
        switch index_max
            case 1 % Red is maximum
                HUE = 60 * ( mod((rgb(2) - rgb(3))/delta, 6) );
            case 2 % Green is maximum
                HUE = 60 * ( (rgb(3) - rgb(1))/delta + 2 );
            case 3 % Blue is maximum
                HUE = 60 * ( (rgb(1) - rgb(2))/delta + 4 );
        end
    end

HUE_360 = HUE;
HUE_255 = HUE*255/360; % standard 255 range Hue

end

== matlab function Interpretation_Unit/pointCloud/Find XY Countour ==
  data: distances input; X output size=720; heading input; Y output size=720; d_max input
function [X, Y] = LIDAR2XY(distances, heading, d_max)

% find indices where distances corresponds to the d_max (bordering circle)
idx = distances < d_max;

% drop the bordering circle
temp_distances = distances(idx);
temp_heading = heading(idx);

% find X, Y pairs from distance, heading
X = temp_distances.*cos(temp_heading);
Y = temp_distances.*sin(temp_heading);

== matlab function Interpretation_Unit/obstacleDetection/Draw Lines Module ==
  data: img_in input; img_out output; pts input; color input
function img_out = drawLines(img_in, pts, color)

% Draw lines connecting the points using the provided color

% Inputs:
% u         : Input RGB Image (size = m by n)
% pts       : p x-y pairs of points (px) where markers are to be drawn
% color     : 1x3 matrix of RGB color values for each marker

% Outputs:
% y         : Output RGB Image with the markers drawn in (size = m by n)

%% Initialization
img_out = img_in;
[p, ~] = size(pts); % determine the number of points

%% Draw the lines
    for i = 1:p-1
        % determine the max(rows_difference, col_difference) between two
        % points
        itr = max(abs(pts(i,1) - pts(i+1,1)), abs(pts(i,2) - pts(i+1,2)));
        
        % generate linear spaces of row and col values between the pts
        row_vec = round(linspace(pts(i,1), pts(i+1,1), itr));
        col_vec = round(linspace(pts(i,2), pts(i+1,2), itr));
        
        % iterate through the values and shade them right
        for j = 1:itr
            img_out(row_vec(j), col_vec(j),1) = color(1);
            img_out(row_vec(j), col_vec(j),2) = color(2);
            img_out(row_vec(j), col_vec(j),3) = color(3);
        end
    end
end

== matlab function Interpretation_Unit/colorCorrectionCSI/MATLAB Function ==
  data: A input; B output; alpha input; beta input
function B = color_correct(A, alpha, beta)

[m, n, p] = size(A);
B = uint8(zeros(m, n, p));

for i = 1:m
    for j = 1:n
        d = ((i - m/2)^2 + (j - n/2)^2)^0.5;
        B(i, j, 1) = uint8(double(A(i, j, 1)) * (1 + beta(1) * exp(-d^2/100000)) * alpha(1));
        B(i, j, 2) = uint8(double(A(i, j, 2)) * (1 - beta(2) * exp(-d^2/100000)) * alpha(2));
        B(i, j, 3) = uint8(double(A(i, j, 3)) * (1 + beta(3) * exp(-d^2/100000)) * alpha(3));
    end
end

== matlab function Interpretation_Unit/pointCloud/Countour to Point Cloud ==
  data: X input [0..720]; map_out output; Y input
function map_out = XYPairs2Map(X, Y)

dim = 400; % Image size will be [dim x dim]
gain = 50; % 50 pixels per meter

persistent map_internal
if isempty(map_internal)
    map_internal = zeros(dim, dim);
else
    map_internal = 0*map_internal; % erase older data... change 0 if you want
end

pX = round(dim/2 - X*gain); % X coordinates w.r.t image center
pY = round(dim/2 - Y*gain); % Y coordinates w.r.t image center

% At the locations corresponding to pX and pY, set a value of 1
map_internal(sub2ind([dim, dim], pX, pY)) = 1;

map_out = map_internal;

== matlab function Interpretation_Unit/linearPolyFit ==
  data: Binary input; m output; b output
function [m, b] = linearPolyFit(Binary)

% find row, col pairs of points where pixel value is bright
[rows, cols] = find(Binary > 0);

% grab sub set of these points randomly
n = length(cols); % total points = n
p = floor(n/3);  % subset of points
        % try p = n/2, or n/3 for 2 or 3 times faster algorithm, etc.

idx = randperm(n, p); % indices corresponding to these

% x is coloumns, y is max_row - rows
x = cols;
y = 150 - rows;

% fit a linear polynomial to the points and grab slope, intercept
result = polyfit(x(idx), y(idx), 1);
m = result(1); 
b = result(2);

== matlab function Interpretation_Unit/obstacleDetection/MATLAB Function ==
  data: depth input; y output; minDistance input; maxDistance input
function y = calculateDistance(depth, minDistance, maxDistance)

% This function drops depth data when outside the minDistance:maxDistance
% bounds and then averages the result. 

u_flat = reshape(depth, 1, []);
u_flat(u_flat < minDistance) = [];
u_flat(u_flat > maxDistance) = [];
y = mean(mean(u_flat));

== matlab function Interpretation_Unit/obstacleDetection/Quick Resize ==
  data: u input; y output
function y = quickResize(u)

scale = 2;
    if length(size(u)) == 3
        y = u(1:scale:end, 1:scale:end, :);
    else
        y = u(1:scale:end, 1:scale:end);
    end

end

== matlab function Interpretation_Unit/obstacleDetection/Steering based image subselector ==
  data: pts output; depth input; region output; steering input
function [pts, region] = drawBox(depth, steering)

mark = 640 - (steering*520/0.5);
starting_index = mark+1-120;
region = double(depth(241:480, starting_index : starting_index + 239));
pts = [ 241, mark+1-120; 241, mark+120; 480, mark+120; 480, mark+1-120; 241, mark+1-120];

== matlab function Interpretation_Unit/intelRealsenseRGB2Depth ==
  data: rgb_coordinates input; depth_coordinates output
function depth_coordinates = rgb720ToDepth720(rgb_coordinates)

% Inputs:
% rgbCoordinates - row, coloumn coordinates of a point in a 1280x720x3 RGB image
% 
% Outputs:
% depthCoordinates - row, coloumn coordinates of a corresponding point in the 1280x720x3 Depth image

depth_coordinates = [-0.0109 *rgb_coordinates(2) + 0.7173 *rgb_coordinates(1) +  93.5549 ,...
                      0.7180 *rgb_coordinates(2) - 0.0041 *rgb_coordinates(1) + 160.3001 ];
